simulink model "ModSim_ex7_1c_model"  (R2016a)
settings: Solver=ode45  StartTime=0.0  StopTime=tsim  RelTol=1e-3
values from neighbouring files (symbols this model uses):
  A = A + diag(v,-1)    [ModSim_ex7_1c_init.m]
  B = zeros(N+N-1,2)    [ModSim_ex7_1c_init.m]
  C = zeros(2,N+N-1)    [ModSim_ex7_1c_init.m]
  D = zeros(2,2)    [ModSim_ex7_1c_init.m]
  x_0 = zeros(N+N-1,1)    [ModSim_ex7_1c_init.m]
settings Model: Creator=camister  LastModifiedBy=camillasterud
settings DataIOCC: LimitDataPoints=on  SaveFormat=Array
settings HardwareCC: ProdBitPerPointer=32  ProdLargestAtomicFloat=None  ProdIntDivRoundTo=Undefined  ProdEndianess=Unspecified  ProdWordSize=32  ProdHWDeviceType=32-bit Generic
settings ModelReferenceCC: PropagateSignalLabelsOutOfModel=off
settings ConfigComp: CovModelRefEnable=Off

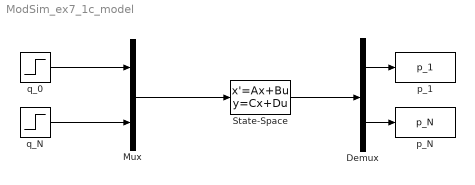
== system ModSim_ex7_1c_model ==
  Demux : Demux  Outputs=2
  Mux : Mux  Inputs=2
  State-Space : StateSpace  A=A  B=B  C=C  D=D  X0=x_0
  p_1 : ToWorkspace  VariableName=p_1  SaveFormat=Timeseries  SampleTime=-1
  p_N : ToWorkspace  VariableName=p_N  SaveFormat=Timeseries  SampleTime=-1
  q_0 : Step  After=0.001  SampleTime=0
  q_N : Step  Time=2  After=0.001  SampleTime=0
  wires:
  State-Space/1 -> Demux/1
  Mux/1 -> State-Space/1
  Demux/1 -> p_1/1
  Demux/2 -> p_N/1
  q_0/1 -> Mux/1
  q_N/1 -> Mux/2
